simulink model "BAI2"  (R2019a)
settings: Solver=ode5  StartTime=0.0  StopTime=10000  FixedStep=1  RelTol=1e-3  EnableMultiTasking=on
undefined symbols (not defined in the file): sigbuilder_block
libraries: fuzblock x1
settings Model: Creator=lemin  LastModifiedBy=forev
settings DataIOCC: LimitDataPoints=on  SaveFormat=Array  SignalLoggingSaveFormat=ModelDataLogs  ReturnWorkspaceOutputs=off
settings OptimizationCC: ExpressionDepthLimit=2147483647  LifeSpan=inf
settings DebuggingCC: UnderspecifiedInitializationDetection=Classic  MergeDetectMultiDrivingBlocksExec=none  SolverPrmCheckMsg=warning  FcnCallInpInsideContextMsg=warning  StateNameClashWarn=warning  SFUnexpectedBacktrackingDiag=warning  SFNoUnconditionalDefaultTransitionDiag=warning  ArithmeticOperatorsInVariantConditions=warning
settings HardwareCC: ProdBitPerPointer=32  ProdBitPerSizeT=32  ProdBitPerPtrDiffT=32  ProdLargestAtomicFloat=None  ProdIntDivRoundTo=Undefined  ProdEndianess=Unspecified  ProdWordSize=32  ProdHWDeviceType=32-bit Generic
settings ModelReferenceCC: PropagateSignalLabelsOutOfModel=off
settings SFSimCC: SimUseLocalCustomCode=off
settings RTWCC: RTWUseLocalCustomCode=off
settings CodeAppCC: StateflowObjectComments=on
settings GRTTargetCC: TargetLangStandard=C89/C90 (ANSI)  GeneratePreprocessorConditionals=Disable all  CombineOutputUpdateFcns=off  GRTInterface=on
settings ConfigComp: CovMetricSettings=dw  CovHtmlReporting=on  CovSaveCumulativeToWorkspaceVar=on  CovSaveSingleToWorkspaceVar=on  CovExternalEMLEnable=off

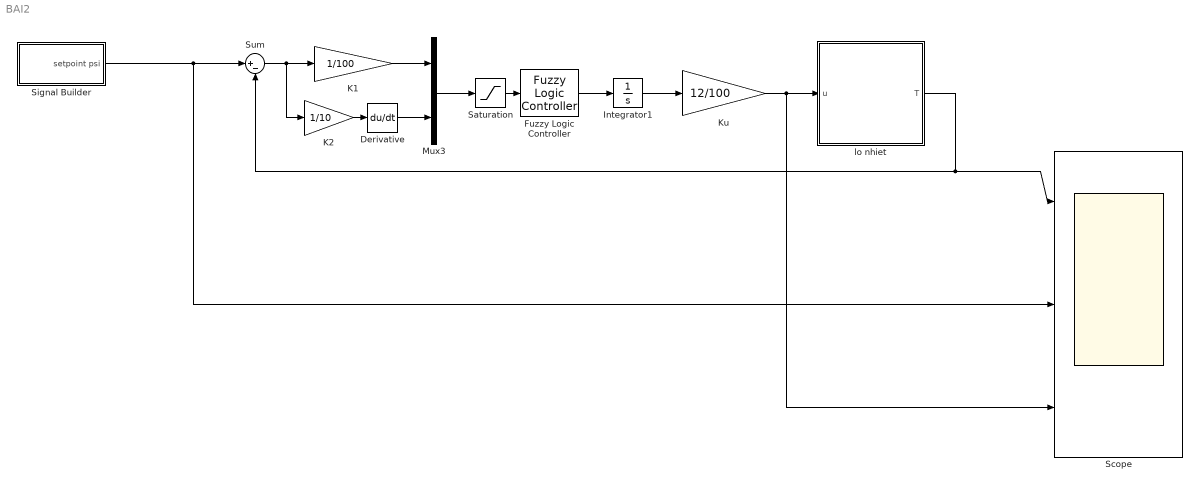
== system BAI2 ==
  Derivative : Derivative
  Fuzzy Logic Controller : fuzblock/Fuzzy Logic  Controller  FIS='PI-lonhiet.fis'  OutputSampleNumber=101  DataType=double  FuzzifiedInputs=off  RuleFiringStrengths=off  RuleOutputs=off  AggregatedOutputs=off  SimulateUsing=Interpreted execution  OutOfRangeInputValueMessage=warning  NoRuleFiredMessage=warning  EmptyOutputFuzzySetMessage=warning
  Integrator1 : Integrator
  "K1 " : Gain  Gain=1/100
  K2 : Gain  Gain=1/10
  Ku : Gain  Gain=12/100
  Mux3 : Mux  Inputs=2
  Saturation : Saturate  UpperLimit=1  LowerLimit=-1
  Scope : Scope  NumInputPorts=3
  Signal Builder : Subsystem  Tag=STV Subsys  LoadFcn=sigbuilder_block('load');  StartFcn=sigbuilder_block('start');  StopFcn=sigbuilder_block('stop');  ClipboardFcn=sigbuilder_block('clipboard');  mask(Sigbuilder block){tuvar=[0:10]}
      mask help: Simulink:masks:SigbuilderBlock_MD
      mask init:
      | if ~strcmp(get_param(bdroot(gcbh),'SimulationStatus'),'stopped') tuvar = sigbuilder_block('maskInit'); end
      settings: CopyFcn=sigbuilder_block('copy');  DeleteFcn=sigbuilder_block('delete');  ModelCloseFcn=sigbuilder_block('modelClose');  PreSaveFcn=sigbuilder_block('preSave');  PauseFcn=sigbuilder_block('pause');  ContinueFcn=sigbuilder_block('continue');  NameChangeFcn=sigbuilder_block('namechange');  OpenFcn=sigbuilder_block('open',[5.4 30 1141.2 522.6 ]);  CloseFcn=sigbuilder_block('close');
      mask Display: plot(0, 0, 100, 100,[2, 2, 32, 32, 2], [68, 8, 8, 68, 68],[32, 2], [38, 38], [32, 19, 2],[53, 60, 44], [32, 17, 17, 2],[16, 16, 31, 31]);txt = getActiveGroup(gcbh);text(2, 100, txt,'verticalAlignment', 'top');
  Sum : Sum  Inputs=|+-
  lo nhiet : Subsystem  mask{l=250, v=8, k=5.88*8/250, t1=-16.91*250/8, t2=0.45*250/8, t3=1.43*250/8, psi3dot0=0, psi2dot0=0, psi1dot0=0}
      mask prompts: l "chieu dai tau"; v "van toc tau"
  wires:
  Ku/1 -> Scope/3, lo nhiet/1("u ")
  Sum/1 -> K2/1, "K1 "/1
  K2/1 -> Derivative/1
  Derivative/1 -> Mux3/2
  "K1 "/1 -> Mux3/1
  lo nhiet/1(T) -> Sum/2, Scope/1
  Saturation/1 -> Fuzzy Logic Controller/1
  Mux3/1 -> Saturation/1
  Signal Builder/1(setpoint psi) -> Scope/2, Sum/1
  Integrator1/1 -> Ku/1
  Fuzzy Logic Controller/1 -> Integrator1/1

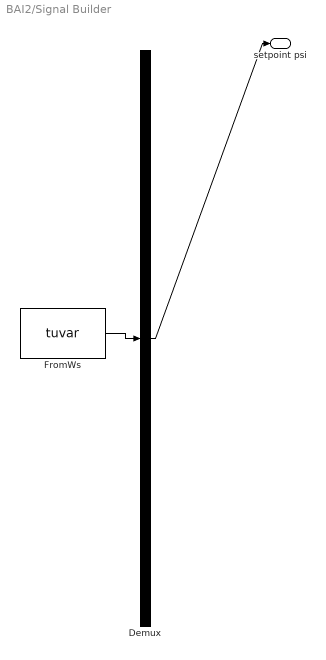
== system BAI2/Signal Builder ==
  Demux : Demux  Tag=STV Demux  Outputs=1
  FromWs : FromWorkspace  Tag=STV FromWs  VariableName=tuvar  SampleTime=0
      SigBuilderData=|
      | common.afterFinalStr = 'Extrapolate'
      | common.sampleTime = 0
      | dataSet.timeRange = [0 1000]
      | dataSet.name = 'Group 1'
      | sbobj.Groups.Name = 'Group 1'
      | sbobj.Groups.Signals.Name = 'setpoint psi'
      | sbobj.Groups.Signals.XData = [0 78 78 1000]
      | sbobj.Groups.Signals.YData = [0 0 191 191]
      | sbobj.Groups.TimeRange = [0 1000]
  setpoint psi : Outport  Tag=STV Outport
  wires:
  FromWs/1 -> Demux/1
  Demux/1 -> setpoint psi/1

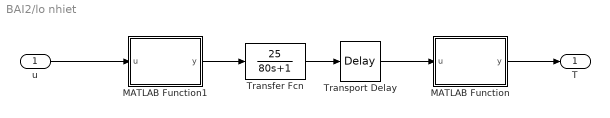
== system BAI2/lo nhiet ==
  "u " : Inport
  MATLAB Function : MATLAB Function  TreatAsAtomicUnit=on
  MATLAB Function1 : MATLAB Function  TreatAsAtomicUnit=on
  Transfer Fcn : TransferFcn  Numerator=[25]  Denominator=[80 1]
  Transport Delay : TransportDelay  DelayTime=20
  T : Outport
  wires:
  Transfer Fcn/1 -> Transport Delay/1
  Transport Delay/1 -> MATLAB Function/1(u)
  MATLAB Function/1(y) -> T/1
  MATLAB Function1/1(y) -> Transfer Fcn/1
  "u "/1 -> MATLAB Function1/1(u)

== matlab function BAI2/lo nhiet/MATLAB Function1 ==
  data: u input; y output
function y = fcn(u)
    if u > 12
        u = 12;
    end
    if u < 0
        u = 0;
    end
y = u;

== matlab function BAI2/lo nhiet/MATLAB Function ==
  data: u input; y output
function y = fcn(u)
    if u > 300
        u = 300;
    end
    
    if u < 0
        u = 0;
    end
y = u;
